simulink model "suraR2012bslx"  (R2012b)
settings: Solver=ode45  StartTime=0.0  StopTime=10  MaxStep=0.0001  RelTol=1e-8
settings Model: CovMetricSettings=dwe  CovHtmlReporting=off  covSaveCumulativeToWorkspaceVar=off  CovSaveSingleToWorkspaceVar=off  CovExternalEMLEnable=on  Creator=user  LastModifiedBy=user
settings DataIOCC: SaveFormat=StructureWithTime  SaveOutput=off  SaveTime=off
settings OptimizationCC: LifeSpan=1
settings DebuggingCC: SolverPrmCheckMsg=none  FcnCallInpInsideContextMsg=EnableAllAsWarning  FrameProcessingCompatibilityMsg=error
settings HardwareCC: ProdBitPerPointer=64  ProdLargestAtomicFloat=Float  ProdIntDivRoundTo=Zero  ProdEndianess=LittleEndian  ProdHWDeviceType=Specified
settings ModelReferenceCC: PropagateSignalLabelsOutOfModel=on
settings CodeAppCC: CustomSymbolStrType=$N$R$M_T
settings GRTTargetCC: CodeReplacementLibrary=C89/C90 (ANSI)  CombineOutputUpdateFcns=off  GRTInterface=on

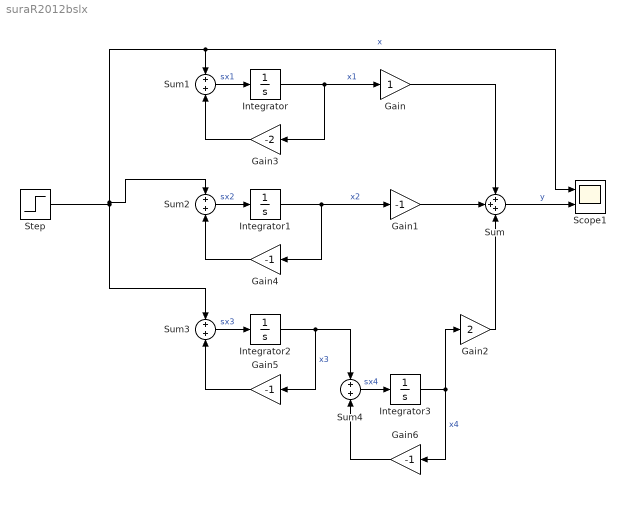
== system suraR2012bslx ==
  Gain : Gain
  Gain{1,4..6} (4 alike) : Gain  Gain=-1
  Gain2 : Gain  Gain=2
  Gain3 : Gain  Gain=-2
  Integrator{,1..3} (4 alike) : Integrator
  Scope1 : Scope  NumInputPorts=2
      settings: ShowLegends=on  YMin=-0.18748~-5  YMax=1.68736~5
  Step : Step  Description=skok jednostkowy  SampleTime=0
  Sum : Sum  Inputs=3
  Sum{1..4} (4 alike) : Sum  Inputs=2
  wires:
  Step/1 -> Sum3/1, Sum2/1, Sum1/1, Scope1/1  "x"
  Sum/1 -> Scope1/2  "y"
  Sum1/1 -> Integrator/1  "sx1"
  Integrator/1 -> Gain3/1, Gain/1  "x1"
  Gain3/1 -> Sum1/2
  Gain4/1 -> Sum2/2
  Sum2/1 -> Integrator1/1  "sx2"
  Integrator1/1 -> Gain4/1, Gain1/1  "x2"
  Sum3/1 -> Integrator2/1  "sx3"
  Gain5/1 -> Sum3/2
  Gain1/1 -> Sum/2
  Gain/1 -> Sum/1
  Gain2/1 -> Sum/3
  Sum4/1 -> Integrator3/1  "sx4"
  Integrator2/1 -> Gain5/1, Sum4/1  "x3"
  Integrator3/1 -> Gain2/1, Gain6/1  "x4"
  Gain6/1 -> Sum4/2
